simulink model "pmsm"  (R2018b)
settings: Solver=FixedStepAuto  StartTime=0.0  StopTime=1  FixedStep=simulation_time_step  RelTol=1e-3
values from neighbouring files (symbols this model uses):
  gamma = 1000    [pmsm_code.m]
  L = (3/2) * 3.752e-4    (= 0.0005628)    [pmsm_code.m]
  phase_frequency_radians = phase_frequency * 2 * pi    (= 62.8318530718)    [pmsm_code.m]
  psi = 0.1194    [pmsm_code.m]
  pwm_frequency = 10000    [pmsm_code.m]
  R = (3/2) * 0.34    (= 0.51)    [pmsm_code.m]
  V = 75    [pmsm_code.m]
libraries: peTransforms x2, autolibpmsmexterior x1
settings Model: Creator=root  LastModifiedBy=skimberk

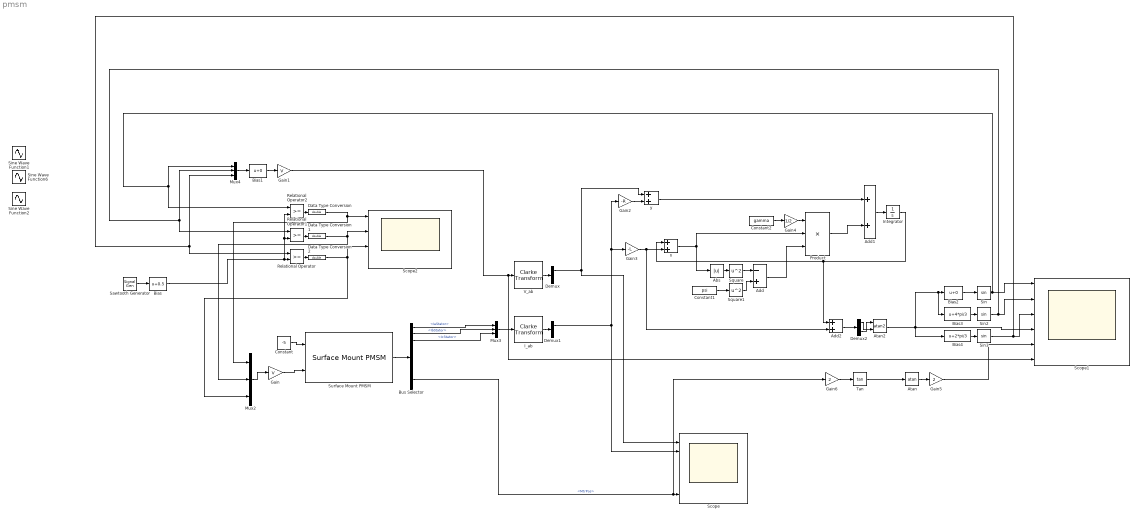
== system pmsm ==
  Abs : Abs
  Add : Sum  Inputs=-+
  Add1 : Sum
  Add2 : Sum
  Atan : Trigonometry  Operator=atan
  Atan2 : Trigonometry  Operator=atan2
  Bias : Bias  Bias=0.5
  Bias1 : Bias
  Bias2 : Bias
  Bias3 : Bias  Bias=4*pi/3
  Bias4 : Bias  Bias=2*pi/3
  Bus Selector : BusSelector  OutputSignals=IaStator,IbStator,IcStator,IdSync,IqSync,VdSync,VqSync,MtrSpd,MtrPos,MtrTrq
  Constant : Constant  Value=-5
  Constant1 : Constant  Value=psi
  Constant2 : Constant  Value=gamma
  Data Type Conversion : DataTypeConversion  OutDataTypeStr=double
  Data Type Conversion1 : DataTypeConversion  OutDataTypeStr=double
  Data Type Conversion2 : DataTypeConversion  OutDataTypeStr=double
  Demux : Demux  Outputs=2
  Demux1 : Demux  Outputs=2
  Demux2 : Demux  Outputs=2
  Gain : Gain  Gain=V
  Gain1 : Gain  Gain=V
  Gain2 : Gain  Gain=-R
  Gain3 : Gain  Gain=-L
  Gain4 : Gain  Gain=1/2
  Gain5 : Gain  Gain=2
  Gain6 : Gain  Gain=2
  I_ab : peTransforms/Clarke Transform  PowerInvariant=off
  Integrator : Integrator
  Mux2 : Mux  Inputs=3
  Mux3 : Mux  Inputs=3
  Mux4 : Mux  Inputs=3
  Product : Product  Inputs=3
  Relational Operator : RelationalOperator  OutDataTypeStr=boolean  RndMeth=Simplest
  Relational Operator1 : RelationalOperator  OutDataTypeStr=boolean  RndMeth=Simplest
  Relational Operator2 : RelationalOperator  OutDataTypeStr=boolean  RndMeth=Simplest
  Sawtooth Generator : SignalGenerator  WaveForm=sawtooth  Amplitude=0.5  Frequency=pwm_frequency
  Scope : Scope  NumInputPorts=7
  Scope1 : Scope  NumInputPorts=6
  Scope2 : Scope  NumInputPorts=4
  Sin : Trigonometry
  Sin2 : Trigonometry
  Sin3 : Trigonometry
  Sine Wave Function1 : Sin  Amplitude=0.5  Bias=0.5  Frequency=phase_frequency_radians  SampleTime=0
  Sine Wave Function2 : Sin  Amplitude=0.5  Bias=0.5  Frequency=phase_frequency_radians  Phase=4*pi/3  SampleTime=0
  Sine Wave Function6 : Sin  Amplitude=0.5  Bias=0.5  Frequency=phase_frequency_radians  Phase=2*pi/3  SampleTime=0
  Square : Math  Operator=square  SaturateOnIntegerOverflow=on
  Square1 : Math  Operator=square  SaturateOnIntegerOverflow=on
  Surface Mount PMSM : autolibpmsmexterior/Surface Mount PMSM  port_config=Torque  Rs=0.54  Ldq_=3.752e-4  lambda_pm=0.1194  P=4  idq0=[0 0]  theta_init=0  omega_init=1000  mechanical=[0.0027, 4.924e-4, 0]  Ldq="[0.0003752   0.0003752]"
      settings: SourceProductName=Powertrain Blockset  SourceProductBaseCode=PW
  Tan : Trigonometry  Operator=tan
  V_ab : peTransforms/Clarke Transform  PowerInvariant=off
  n : Sum
  y : Sum
  wires:
  Surface Mount PMSM/1 -> Bus Selector/1
  Constant/1 -> Surface Mount PMSM/1
  Gain/1 -> Surface Mount PMSM/2
  Sawtooth Generator/1 -> Bias/1
  Sin3/1 -> Relational Operator/1, Mux4/3, Scope1/3
  Bias/1 -> Relational Operator1/2, Relational Operator2/2, Relational Operator/2
  Sin2/1 -> Relational Operator1/1, Mux4/2, Scope1/2
  Sin/1 -> Relational Operator2/1, Mux4/1, Scope1/1
  Mux2/1 -> Gain/1
  Relational Operator2/1 -> Data Type Conversion/1
  Relational Operator1/1 -> Data Type Conversion1/1
  Relational Operator/1 -> Data Type Conversion2/1
  Data Type Conversion/1 -> Mux2/1, Scope2/1
  Data Type Conversion1/1 -> Scope2/2, Mux2/2
  Data Type Conversion2/1 -> Mux2/3, Scope2/3
  Bus Selector/1 -> Mux3/1  "<IaStator>"
  Bus Selector/2 -> Mux3/2  "<IbStator>"
  Bus Selector/3 -> Mux3/3  "<IcStator>"
  Mux3/1 -> I_ab/1
  Bus Selector/9 -> Gain6/1, Scope/7  "<MtrPos>"
  Mux4/1 -> Bias1/1
  Gain1/1 -> Scope1/6, V_ab/1
  Bias1/1 -> Gain1/1
  Demux1/1 -> Scope/2, Gain3/1, Gain2/1
  Demux/1 -> Scope/1, y/1
  Gain2/1 -> y/2
  Gain3/1 -> n/2, Add2/2
  Abs/1 -> Square/1
  n/1 -> Abs/1, Product/2
  Square/1 -> Add/1
  Constant1/1 -> Square1/1
  Add/1 -> Product/3
  y/1 -> Add1/1
  Product/1 -> Add1/2
  Constant2/1 -> Gain4/1
  Gain4/1 -> Product/1
  Square1/1 -> Add/2
  Add1/1 -> Integrator/1
  Integrator/1 -> Add2/1, n/1
  V_ab/1 -> Demux/1
  I_ab/1 -> Demux1/1
  Add2/1 -> Demux2/1
  Demux2/2 -> Atan2/1
  Demux2/1 -> Atan2/2
  Bias2/1 -> Sin/1
  Bias3/1 -> Sin2/1
  Bias4/1 -> Sin3/1
  Atan2/1 -> Bias4/1, Bias3/1, Bias2/1, Scope1/4
  Gain6/1 -> Tan/1
  Atan/1 -> Gain5/1
  Tan/1 -> Atan/1
  Gain5/1 -> Scope1/5
